simulink model "state1"  (Simulink 9.0)
settings: Solver=ode45  StartTime=0.0  StopTime=TMax  RelTol=1e-3  EnableMultiTasking=on
values from neighbouring files (symbols this model uses):
  alpha = exp(-2*pi*DT*fc)    [1_state.m]
  DT = 0.01    [1_state.m]
  G = -place(A,B,pole)    [1_state.m]
  PC_MaxPit = 1.570796    [1_state.m]
  PC_MaxRat = 0.1396263    [1_state.m]
  PC_MinPit = 0.0    (= 0)    [1_state.m]
  ref_pitch = 7.06205E-02    (= 0.0706205)    [1_state.m]
  ref_rot = 1.2671090354999999    (= 1.2671090355)    [1_state.m]
undefined symbols (not defined in the file or in its folder): OutList, strmatch
libraries: simulink_extras x1
settings Model: Creator=Avell 1513  LastModifiedBy=Avell 1513
settings DataIOCC: LimitDataPoints=on
settings DebuggingCC: SolverPrmCheckMsg=warning  StateNameClashWarn=warning
settings GRTTargetCC: GeneratePreprocessorConditionals=Disable all

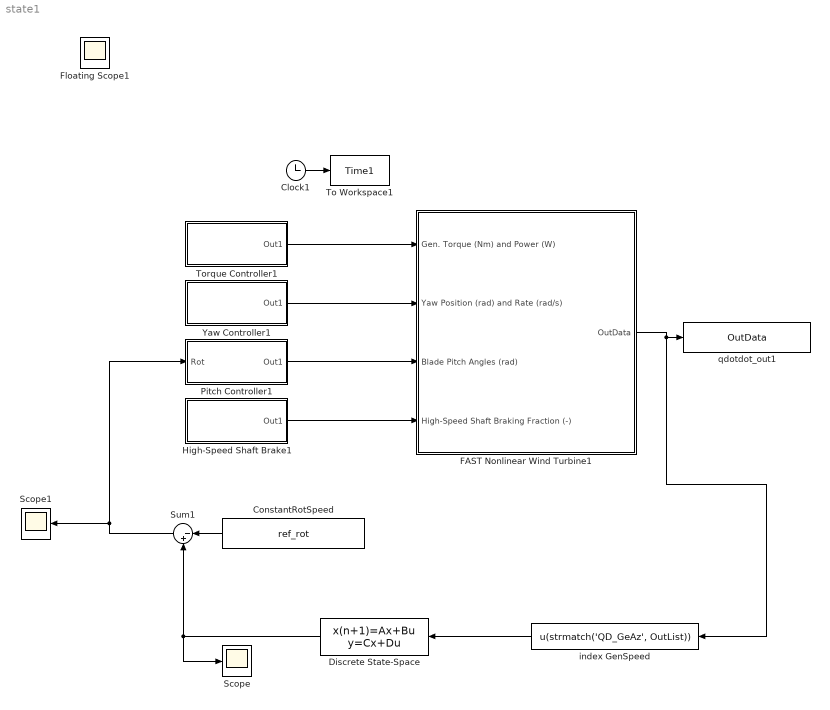
== system state1 ==
  Clock1 : Clock
  ConstantRotSpeed : Constant  Value=ref_rot
  Discrete State-Space : DiscreteStateSpace  A=alpha  B=1-alpha  C=alpha  D=1-alpha  InitialCondition=ref_rot  SampleTime=DT
  FAST Nonlinear Wind Turbine1 : Subsystem  mask(FAST Nonlinear Wind Turbine){}
      mask help: This block contains the FAST S-Function.
      mask init:
      | clear FAST_SFunc
  High-Speed Shaft Brake1 : Subsystem
  Pitch Controller1 : Subsystem
  Scope : Scope
  Scope1 : Scope
  Sum1 : Sum  Inputs=|-+
  To Workspace1 : ToWorkspace  VariableName=Time1  SampleTime=-1
  Torque Controller1 : Subsystem
  Yaw Controller1 : Subsystem
  index GenSpeed : Fcn  Expr=u(strmatch('QD_GeAz', OutList))
  qdotdot_out1 : ToWorkspace  VariableName=OutData  SampleTime=-1
  Floating Scope1 : Scope
  wires:
  ConstantRotSpeed/1 -> Sum1/1
  Sum1/1 -> Pitch Controller1/1(Rot), Scope1/1
  FAST Nonlinear Wind Turbine1/1(OutData) -> index GenSpeed/1, qdotdot_out1/1
  Yaw Controller1/1(Out1) -> FAST Nonlinear Wind Turbine1/2(Yaw Position (rad) and Rate (rad/s))
  Pitch Controller1/1(Out1) -> FAST Nonlinear Wind Turbine1/3(Blade Pitch Angles (rad))
  High-Speed Shaft Brake1/1(Out1) -> FAST Nonlinear Wind Turbine1/4(High-Speed Shaft Braking Fraction (-))
  Clock1/1 -> To Workspace1/1
  Torque Controller1/1(Out1) -> FAST Nonlinear Wind Turbine1/1(Gen. Torque (Nm) and Power (W))
  Discrete State-Space/1 -> Sum1/2, Scope/1
  index GenSpeed/1 -> Discrete State-Space/1

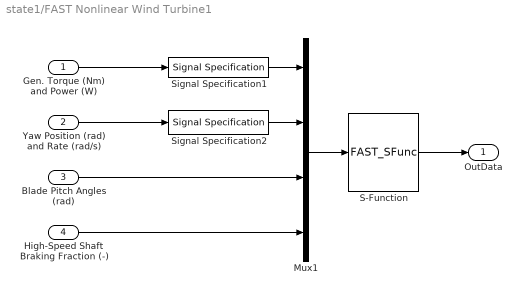
== system state1/FAST Nonlinear Wind Turbine1 ==
  Gen. Torque (Nm) and Power (W) : Inport
  Yaw Position (rad) and Rate (rad/s) : Inport  Port=2
  Blade Pitch Angles (rad) : Inport  Port=3
  High-Speed Shaft Braking Fraction (-) : Inport  Port=4
  Mux1 : Mux
  S-Function : S-Function  FunctionName=FAST_SFunc  Parameters=FAST_InputFileName, TMax, 0  SFunctionDeploymentMode=off  EnableBusSupport=off
  Signal Specification1 : SignalSpecification  OutDataTypeStr=double  Dimensions=2
  Signal Specification2 : SignalSpecification  OutDataTypeStr=double  Dimensions=2
  OutData : Outport
  wires:
  Gen. Torque (Nm) and Power (W)/1 -> Signal Specification1/1
  S-Function/1 -> OutData/1
  Mux1/1 -> S-Function/1
  Blade Pitch Angles (rad)/1 -> Mux1/3
  Yaw Position (rad) and Rate (rad/s)/1 -> Signal Specification2/1
  Signal Specification1/1 -> Mux1/1
  Signal Specification2/1 -> Mux1/2
  High-Speed Shaft Braking Fraction (-)/1 -> Mux1/4

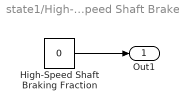
== system state1/High-Speed Shaft Brake1 ==
  High-Speed Shaft Braking Fraction : Constant  Value=0
  Out1 : Outport
  wires:
  High-Speed Shaft Braking Fraction/1 -> Out1/1

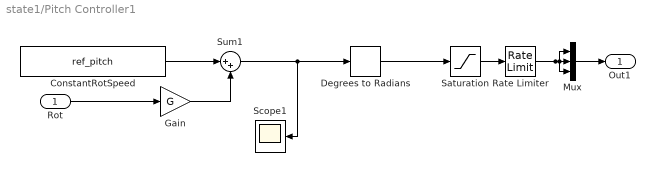
== system state1/Pitch Controller1 ==
  Rot : Inport
  ConstantRotSpeed : Constant  Value=ref_pitch
  Degrees to Radians : simulink_extras/Transformations/Degrees to Radians
  Gain : Gain  Gain=G
  Mux : Mux  Inputs=3
  Rate Limiter : RateLimiter  RisingSlewLimit=PC_MaxRat  FallingSlewLimit=-PC_MaxRat  SampleTimeMode=inherited
  Saturation : Saturate  UpperLimit=PC_MaxPit  LowerLimit=PC_MinPit
  Scope1 : Scope
  Sum1 : Sum  Inputs=|++
  Out1 : Outport
  wires:
  Mux/1 -> Out1/1
  Saturation/1 -> Rate Limiter/1
  Rate Limiter/1 -> Mux/3, Mux/1, Mux/2
  Degrees to Radians/1 -> Saturation/1
  Sum1/1 -> Scope1/1, Degrees to Radians/1
  ConstantRotSpeed/1 -> Sum1/1
  Rot/1 -> Gain/1
  Gain/1 -> Sum1/2

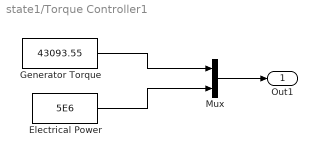
== system state1/Torque Controller1 ==
  Electrical Power : Constant  Value=5E6
  Generator Torque : Constant  Value=43093.55
  Mux : Mux  Inputs=2
  Out1 : Outport
  wires:
  Mux/1 -> Out1/1
  Generator Torque/1 -> Mux/1
  Electrical Power/1 -> Mux/2

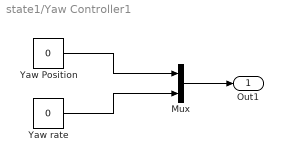
== system state1/Yaw Controller1 ==
  Mux : Mux  Inputs=2
  Yaw Position : Constant  Value=0
  Yaw rate : Constant  Value=0
  Out1 : Outport
  wires:
  Mux/1 -> Out1/1
  Yaw Position/1 -> Mux/1
  Yaw rate/1 -> Mux/2
